simulink model "Leds"  (R2023b)
settings: Solver=VariableStepAuto  StartTime=0.0  StopTime=inf  RelTol=1e-3
libraries: arduinolib x1, simulink x1
settings Model: Creator=Usuario_UMA  LastModifiedBy=alumnos

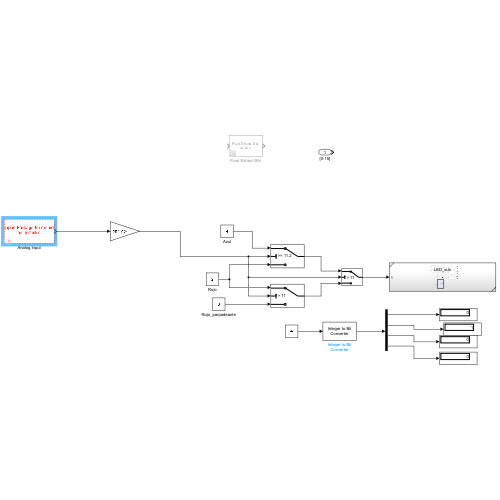
[thumbnail: Simulink's stored preview of the top-level diagram]
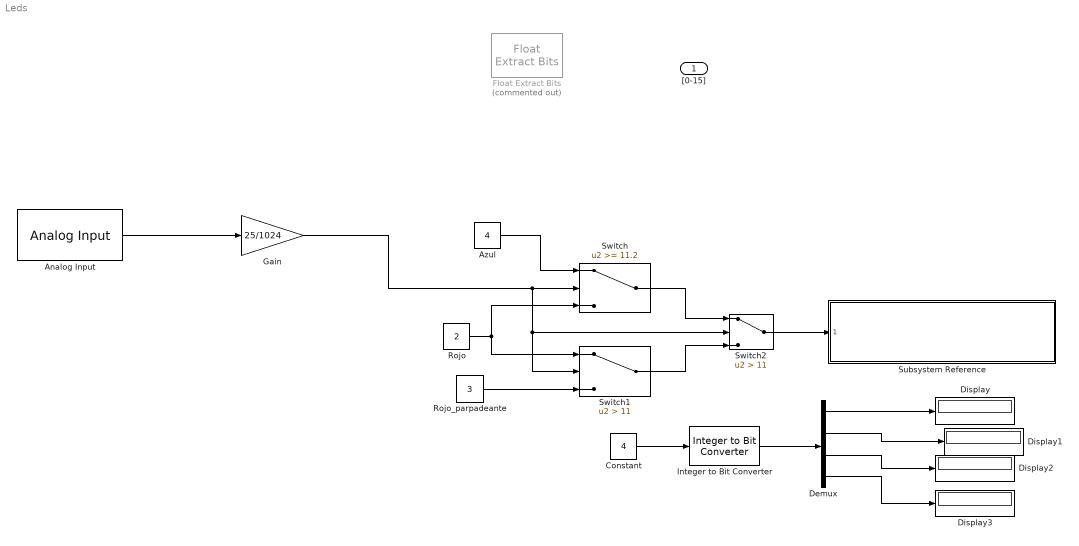
== system Leds ==
  "[0-15]" : Inport
  Analog Input : arduinolib/Analog Input  pinNumber=4  ReadResultsOnly=off  ConversionTriggerSource=Software  ExternalTriggerType=uint32( 0 )  OutputDataType=uint16  EnableConversionCompleteNotify=off  EnableOuputStatus=off  SampleTime=-1  blockPlatform=arduino
  Azul : Constant  Value=4
  Constant : Constant  Value=4
  Demux : Demux
  Display{,1..3} (4 alike) : Display
  Float Extract Bits : FloatExtractBits  Commented=on
  Gain : Gain  Gain=25/1024
  Integer to Bit Converter : simulink/Logic and Bit Operations/Integer to Bit Converter  nbits=4  signedInputValues=Unsigned  bitOrder=MSB first  outDtype=Inherit via internal rule
  Rojo : Constant  Value=2
  Rojo_parpadeante : Constant  Value=3
  Subsystem Reference : Subsystem  ReferencedSubsystem=LED_sub
  Switch : Switch  Threshold=11.2  SaturateOnIntegerOverflow=off  InputSameDT=off
  Switch1 : Switch  Criteria=u2 > Threshold  Threshold=11  SaturateOnIntegerOverflow=off  InputSameDT=off
  Switch2 : Switch  Criteria=u2 > Threshold  Threshold=11  SaturateOnIntegerOverflow=off  InputSameDT=off
  wires:
  Azul/1 -> Switch/1
  Constant/1 -> Integer to Bit Converter/1
  Integer to Bit Converter/1 -> Demux/1
  Demux/1 -> Display/1
  Demux/2 -> Display1/1
  Demux/3 -> Display2/1
  Demux/4 -> Display3/1
  Rojo/1 -> Switch1/1, Switch/3
  Rojo_parpadeante/1 -> Switch1/3
  Switch/1 -> Switch2/1
  Switch1/1 -> Switch2/3
  Switch2/1 -> Subsystem Reference/1
  Analog Input/1 -> Gain/1
  Gain/1 -> Switch2/2, Switch1/2, Switch/2
